simulink subsystem "tcp_trace_simscape_ref_subsys"  (R2022b)
settings: Solver=VariableStepAuto  StartTime=0.0  StopTime=10.0  RelTol=1e-3
undefined symbols (not defined in the file): param_vis
libraries: nesl_utility x300, sm_lib x200
(part 1 of 3)
settings Model: Creator=emu  LastModifiedBy=emu

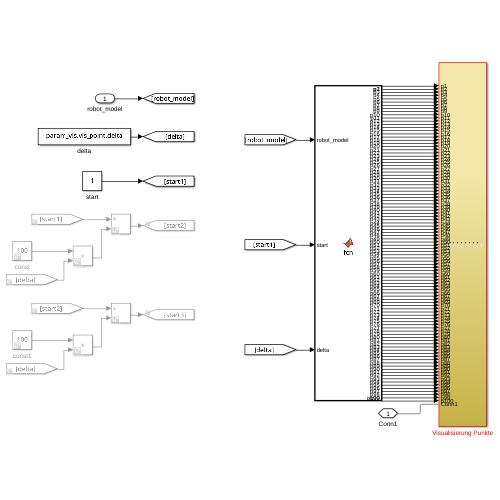
[thumbnail: Simulink's stored preview of the top-level diagram]
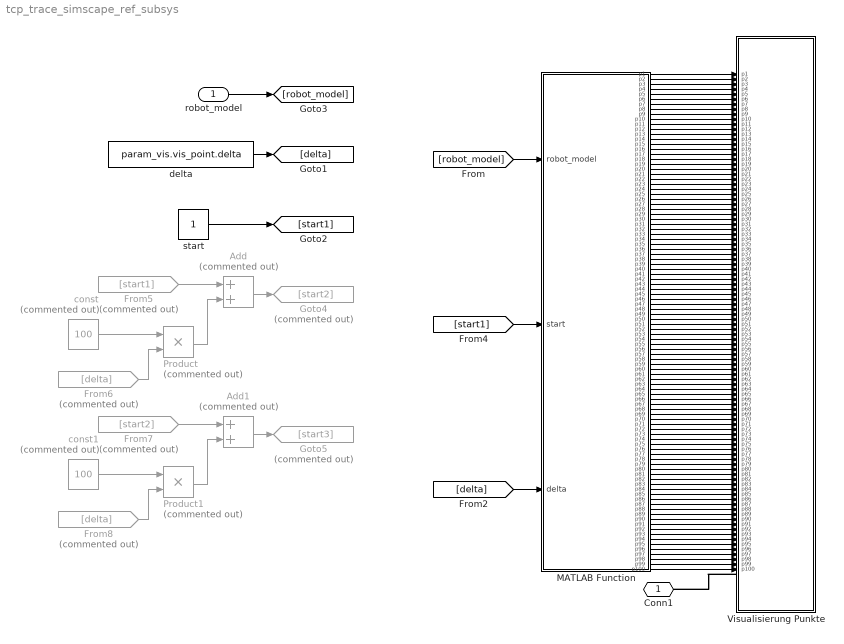
== system tcp_trace_simscape_ref_subsys ==
  robot_model : Inport
  Add : Sum  Commented=on
  Add1 : Sum  Commented=on
  From5 : From  Commented=on  GotoTag=start1
  From6 : From  Commented=on  GotoTag=delta
  From7 : From  Commented=on  GotoTag=start2
  From8 : From  Commented=on  GotoTag=delta
  Goto4 : Goto  Commented=on  GotoTag=start2
  Goto5 : Goto  Commented=on  GotoTag=start3
  MATLAB Function : MATLAB Function  TreatAsAtomicUnit=on
  Product : Product  Commented=on
  Product1 : Product  Commented=on
  Visualisierung Punkte : Subsystem
  const : Constant  Commented=on  Value=100
  const1 : Constant  Commented=on  Value=100
  delta : Constant  Value=param_vis.vis_point.delta
  start : Constant  SampleTime=-1
  Conn1 : PMIOPort  Side=Left
  wires:
  const1/1 -> Product1/1
  MATLAB Function/49(p49) -> Visualisierung Punkte/49(p49)
  Product1/1 -> Add1/2
  MATLAB Function/52(p52) -> Visualisierung Punkte/52(p52)
  MATLAB Function/98(p98) -> Visualisierung Punkte/98(p98)
  MATLAB Function/39(p39) -> Visualisierung Punkte/39(p39)
  MATLAB Function/19(p19) -> Visualisierung Punkte/19(p19)
  MATLAB Function/29(p29) -> Visualisierung Punkte/29(p29)
  MATLAB Function/24(p24) -> Visualisierung Punkte/24(p24)
  MATLAB Function/34(p34) -> Visualisierung Punkte/34(p34)
  MATLAB Function/40(p40) -> Visualisierung Punkte/40(p40)
  MATLAB Function/99(p99) -> Visualisierung Punkte/99(p99)
  MATLAB Function/20(p20) -> Visualisierung Punkte/20(p20)
  From7/1 -> Add1/1
  MATLAB Function/2(p2) -> Visualisierung Punkte/2(p2)
  MATLAB Function/74(p74) -> Visualisierung Punkte/74(p74)
  MATLAB Function/82(p82) -> Visualisierung Punkte/82(p82)
  MATLAB Function/30(p30) -> Visualisierung Punkte/30(p30)
  MATLAB Function/35(p35) -> Visualisierung Punkte/35(p35)
  MATLAB Function/25(p25) -> Visualisierung Punkte/25(p25)
  MATLAB Function/83(p83) -> Visualisierung Punkte/83(p83)
  MATLAB Function/57(p57) -> Visualisierung Punkte/57(p57)
  MATLAB Function/63(p63) -> Visualisierung Punkte/63(p63)
  MATLAB Function/41(p41) -> Visualisierung Punkte/41(p41)
  MATLAB Function/21(p21) -> Visualisierung Punkte/21(p21)
  MATLAB Function/100(p100) -> Visualisierung Punkte/100(p100)
  MATLAB Function/36(p36) -> Visualisierung Punkte/36(p36)
  MATLAB Function/26(p26) -> Visualisierung Punkte/26(p26)
  MATLAB Function/31(p31) -> Visualisierung Punkte/31(p31)
  MATLAB Function/17(p17) -> Visualisierung Punkte/17(p17)
  MATLAB Function/6(p6) -> Visualisierung Punkte/6(p6)
  MATLAB Function/46(p46) -> Visualisierung Punkte/46(p46)
  MATLAB Function/37(p37) -> Visualisierung Punkte/37(p37)
  MATLAB Function/32(p32) -> Visualisierung Punkte/32(p32)
  MATLAB Function/27(p27) -> Visualisierung Punkte/27(p27)
  [delta] -> MATLAB Function/3(delta)
  MATLAB Function/42(p42) -> Visualisierung Punkte/42(p42)
  MATLAB Function/22(p22) -> Visualisierung Punkte/22(p22)
  MATLAB Function/85(p85) -> Visualisierung Punkte/85(p85)
  MATLAB Function/67(p67) -> Visualisierung Punkte/67(p67)
  MATLAB Function/92(p92) -> Visualisierung Punkte/92(p92)
  MATLAB Function/11(p11) -> Visualisierung Punkte/11(p11)
  [start1] -> MATLAB Function/2(start)
  delta/1 -> [delta]
  MATLAB Function/10(p10) -> Visualisierung Punkte/10(p10)
  MATLAB Function/54(p54) -> Visualisierung Punkte/54(p54)
  MATLAB Function/86(p86) -> Visualisierung Punkte/86(p86)
  MATLAB Function/77(p77) -> Visualisierung Punkte/77(p77)
  MATLAB Function/16(p16) -> Visualisierung Punkte/16(p16)
  MATLAB Function/53(p53) -> Visualisierung Punkte/53(p53)
  From8/1 -> Product1/2
  MATLAB Function/38(p38) -> Visualisierung Punkte/38(p38)
  MATLAB Function/33(p33) -> Visualisierung Punkte/33(p33)
  MATLAB Function/28(p28) -> Visualisierung Punkte/28(p28)
  MATLAB Function/23(p23) -> Visualisierung Punkte/23(p23)
  MATLAB Function/59(p59) -> Visualisierung Punkte/59(p59)
  MATLAB Function/91(p91) -> Visualisierung Punkte/91(p91)
  From5/1 -> Add/1
  MATLAB Function/75(p75) -> Visualisierung Punkte/75(p75)
  MATLAB Function/73(p73) -> Visualisierung Punkte/73(p73)
  MATLAB Function/44(p44) -> Visualisierung Punkte/44(p44)
  MATLAB Function/4(p4) -> Visualisierung Punkte/4(p4)
  Add/1 -> Goto4/1
  MATLAB Function/97(p97) -> Visualisierung Punkte/97(p97)
  MATLAB Function/43(p43) -> Visualisierung Punkte/43(p43)
  MATLAB Function/18(p18) -> Visualisierung Punkte/18(p18)
  MATLAB Function/65(p65) -> Visualisierung Punkte/65(p65)
  MATLAB Function/81(p81) -> Visualisierung Punkte/81(p81)
  MATLAB Function/56(p56) -> Visualisierung Punkte/56(p56)
  MATLAB Function/72(p72) -> Visualisierung Punkte/72(p72)
  MATLAB Function/45(p45) -> Visualisierung Punkte/45(p45)
  MATLAB Function/5(p5) -> Visualisierung Punkte/5(p5)
  MATLAB Function/93(p93) -> Visualisierung Punkte/93(p93)
  Product/1 -> Add/2
  MATLAB Function/62(p62) -> Visualisierung Punkte/62(p62)
  const/1 -> Product/1
  MATLAB Function/78(p78) -> Visualisierung Punkte/78(p78)
  MATLAB Function/1(p1) -> Visualisierung Punkte/1(p1)
  From6/1 -> Product/2
  MATLAB Function/47(p47) -> Visualisierung Punkte/47(p47)
  MATLAB Function/7(p7) -> Visualisierung Punkte/7(p7)
  MATLAB Function/79(p79) -> Visualisierung Punkte/79(p79)
  MATLAB Function/9(p9) -> Visualisierung Punkte/9(p9)
  [robot_model] -> MATLAB Function/1(robot_model)
  MATLAB Function/88(p88) -> Visualisierung Punkte/88(p88)
  MATLAB Function/14(p14) -> Visualisierung Punkte/14(p14)
  MATLAB Function/66(p66) -> Visualisierung Punkte/66(p66)
  MATLAB Function/69(p69) -> Visualisierung Punkte/69(p69)
  MATLAB Function/12(p12) -> Visualisierung Punkte/12(p12)
  start/1 -> [start1]
  MATLAB Function/87(p87) -> Visualisierung Punkte/87(p87)
  MATLAB Function/50(p50) -> Visualisierung Punkte/50(p50)
  MATLAB Function/96(p96) -> Visualisierung Punkte/96(p96)
  MATLAB Function/90(p90) -> Visualisierung Punkte/90(p90)
  MATLAB Function/58(p58) -> Visualisierung Punkte/58(p58)
  MATLAB Function/89(p89) -> Visualisierung Punkte/89(p89)
  MATLAB Function/48(p48) -> Visualisierung Punkte/48(p48)
  MATLAB Function/8(p8) -> Visualisierung Punkte/8(p8)
  robot_model/1 -> [robot_model]
  MATLAB Function/13(p13) -> Visualisierung Punkte/13(p13)
  MATLAB Function/80(p80) -> Visualisierung Punkte/80(p80)
  MATLAB Function/70(p70) -> Visualisierung Punkte/70(p70)
  MATLAB Function/15(p15) -> Visualisierung Punkte/15(p15)
  MATLAB Function/3(p3) -> Visualisierung Punkte/3(p3)
  MATLAB Function/84(p84) -> Visualisierung Punkte/84(p84)
  MATLAB Function/76(p76) -> Visualisierung Punkte/76(p76)
  Add1/1 -> Goto5/1
  MATLAB Function/95(p95) -> Visualisierung Punkte/95(p95)
  MATLAB Function/94(p94) -> Visualisierung Punkte/94(p94)
  MATLAB Function/71(p71) -> Visualisierung Punkte/71(p71)
  MATLAB Function/55(p55) -> Visualisierung Punkte/55(p55)
  MATLAB Function/61(p61) -> Visualisierung Punkte/61(p61)
  MATLAB Function/64(p64) -> Visualisierung Punkte/64(p64)
  MATLAB Function/68(p68) -> Visualisierung Punkte/68(p68)
  MATLAB Function/60(p60) -> Visualisierung Punkte/60(p60)
  MATLAB Function/51(p51) -> Visualisierung Punkte/51(p51)
  connections:
  Visualisierung Punkte/LConn1 -- Conn1/RConn1

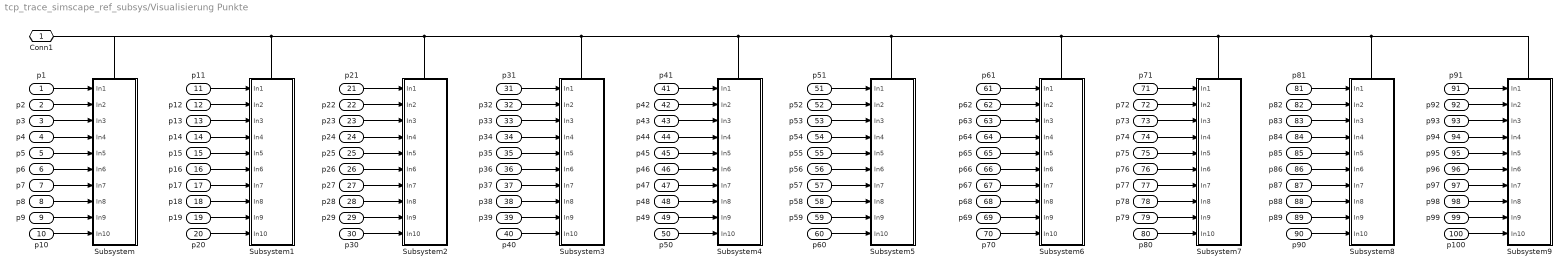
== system tcp_trace_simscape_ref_subsys/Visualisierung Punkte ==
  p1 : Inport
  p2 : Inport  Port=2
  p3 : Inport  Port=3
  p4 : Inport  Port=4
  p5 : Inport  Port=5
  p6 : Inport  Port=6
  p7 : Inport  Port=7
  p8 : Inport  Port=8
  p9 : Inport  Port=9
  p10 : Inport  Port=10
  p11 : Inport  Port=11
  p12 : Inport  Port=12
  p13 : Inport  Port=13
  p14 : Inport  Port=14
  p15 : Inport  Port=15
  p16 : Inport  Port=16
  p17 : Inport  Port=17
  p18 : Inport  Port=18
  p19 : Inport  Port=19
  p20 : Inport  Port=20
  p21 : Inport  Port=21
  p22 : Inport  Port=22
  p23 : Inport  Port=23
  p24 : Inport  Port=24
  p25 : Inport  Port=25
  p26 : Inport  Port=26
  p27 : Inport  Port=27
  p28 : Inport  Port=28
  p29 : Inport  Port=29
  p30 : Inport  Port=30
  p31 : Inport  Port=31
  p32 : Inport  Port=32
  p33 : Inport  Port=33
  p34 : Inport  Port=34
  p35 : Inport  Port=35
  p36 : Inport  Port=36
  p37 : Inport  Port=37
  p38 : Inport  Port=38
  p39 : Inport  Port=39
  p40 : Inport  Port=40
  p41 : Inport  Port=41
  p42 : Inport  Port=42
  p43 : Inport  Port=43
  p44 : Inport  Port=44
  p45 : Inport  Port=45
  p46 : Inport  Port=46
  p47 : Inport  Port=47
  p48 : Inport  Port=48
  p49 : Inport  Port=49
  p50 : Inport  Port=50
  p51 : Inport  Port=51
  p52 : Inport  Port=52
  p53 : Inport  Port=53
  p54 : Inport  Port=54
  p55 : Inport  Port=55
  p56 : Inport  Port=56
  p57 : Inport  Port=57
  p58 : Inport  Port=58
  p59 : Inport  Port=59
  p60 : Inport  Port=60
  p61 : Inport  Port=61
  p62 : Inport  Port=62
  p63 : Inport  Port=63
  p64 : Inport  Port=64
  p65 : Inport  Port=65
  p66 : Inport  Port=66
  p67 : Inport  Port=67
  p68 : Inport  Port=68
  p69 : Inport  Port=69
  p70 : Inport  Port=70
  p71 : Inport  Port=71
  p72 : Inport  Port=72
  p73 : Inport  Port=73
  p74 : Inport  Port=74
  p75 : Inport  Port=75
  p76 : Inport  Port=76
  p77 : Inport  Port=77
  p78 : Inport  Port=78
  p79 : Inport  Port=79
  p80 : Inport  Port=80
  p81 : Inport  Port=81
  p82 : Inport  Port=82
  p83 : Inport  Port=83
  p84 : Inport  Port=84
  p85 : Inport  Port=85
  p86 : Inport  Port=86
  p87 : Inport  Port=87
  p88 : Inport  Port=88
  p89 : Inport  Port=89
  p90 : Inport  Port=90
  p91 : Inport  Port=91
  p92 : Inport  Port=92
  p93 : Inport  Port=93
  p94 : Inport  Port=94
  p95 : Inport  Port=95
  p96 : Inport  Port=96
  p97 : Inport  Port=97
  p98 : Inport  Port=98
  p99 : Inport  Port=99
  p100 : Inport  Port=100
  Subsystem : Subsystem
      settings: PortSchema="{\"entries\":[{\"content\":{\"sides\":[{\"content\":{\"connectorIds\":[\"In1\",\"In2\",\"In3\",\"In4\",\"In5\",\"In6\",\"In7\",\"In8\",\"In9\",\"In10\"]},\"type\":\"ConnectorPlacement.EquallySpacedRectSide\",\"uuid\":\"2018066b-9524-48da-bbe6-ab202b76f720\"},{\"content\":{\"side\":\"RIGHT\"},\"type\":\"ConnectorPlacement.EquallySpacedRectSide\",\"uuid\":\"1983d9d9-cacf-48d4-9900-c1ea83df5447\"},{\"content\":{\"connectorIds\":[\"LConn1\"],\"side\":\"TOP\"},\"type\":\"ConnectorPlacement.EquallySpacedRectSide\",\"uuid\":\"d1112f51-9d46-44e1-99fb-55e38b45bdaf\"}]},\"type\":\"ConnectorPlacement.EquallySpacedConnector\",\"uuid\":\"be633077-5bce-4072-a8b6-d4330dd62166\"}],\"packageUris\":[\"http://schema.mathworks.com/mf0/Connector/R2020b\"],\"version\":\"1.0\"}"
  Subsystem1 : Subsystem
      settings: PortSchema="{\"entries\":[{\"content\":{\"sides\":[{\"content\":{\"connectorIds\":[\"In1\",\"In2\",\"In3\",\"In4\",\"In5\",\"In6\",\"In7\",\"In8\",\"In9\",\"In10\"]},\"type\":\"ConnectorPlacement.EquallySpacedRectSide\",\"uuid\":\"2018066b-9524-48da-bbe6-ab202b76f720\"},{\"content\":{\"side\":\"RIGHT\"},\"type\":\"ConnectorPlacement.EquallySpacedRectSide\",\"uuid\":\"1983d9d9-cacf-48d4-9900-c1ea83df5447\"},{\"content\":{\"connectorIds\":[\"LConn1\"],\"side\":\"TOP\"},\"type\":\"ConnectorPlacement.EquallySpacedRectSide\",\"uuid\":\"d1112f51-9d46-44e1-99fb-55e38b45bdaf\"}]},\"type\":\"ConnectorPlacement.EquallySpacedConnector\",\"uuid\":\"be633077-5bce-4072-a8b6-d4330dd62166\"}],\"packageUris\":[\"http://schema.mathworks.com/mf0/Connector/R2020b\"],\"version\":\"1.0\"}"
  Subsystem2 : Subsystem
      settings: PortSchema="{\"entries\":[{\"content\":{\"sides\":[{\"content\":{\"connectorIds\":[\"In1\",\"In2\",\"In3\",\"In4\",\"In5\",\"In6\",\"In7\",\"In8\",\"In9\",\"In10\"]},\"type\":\"ConnectorPlacement.EquallySpacedRectSide\",\"uuid\":\"2018066b-9524-48da-bbe6-ab202b76f720\"},{\"content\":{\"side\":\"RIGHT\"},\"type\":\"ConnectorPlacement.EquallySpacedRectSide\",\"uuid\":\"1983d9d9-cacf-48d4-9900-c1ea83df5447\"},{\"content\":{\"connectorIds\":[\"LConn1\"],\"side\":\"TOP\"},\"type\":\"ConnectorPlacement.EquallySpacedRectSide\",\"uuid\":\"d1112f51-9d46-44e1-99fb-55e38b45bdaf\"}]},\"type\":\"ConnectorPlacement.EquallySpacedConnector\",\"uuid\":\"be633077-5bce-4072-a8b6-d4330dd62166\"}],\"packageUris\":[\"http://schema.mathworks.com/mf0/Connector/R2020b\"],\"version\":\"1.0\"}"
  Subsystem3 : Subsystem
      settings: PortSchema="{\"entries\":[{\"content\":{\"sides\":[{\"content\":{\"connectorIds\":[\"In1\",\"In2\",\"In3\",\"In4\",\"In5\",\"In6\",\"In7\",\"In8\",\"In9\",\"In10\"]},\"type\":\"ConnectorPlacement.EquallySpacedRectSide\",\"uuid\":\"2018066b-9524-48da-bbe6-ab202b76f720\"},{\"content\":{\"side\":\"RIGHT\"},\"type\":\"ConnectorPlacement.EquallySpacedRectSide\",\"uuid\":\"1983d9d9-cacf-48d4-9900-c1ea83df5447\"},{\"content\":{\"connectorIds\":[\"LConn1\"],\"side\":\"TOP\"},\"type\":\"ConnectorPlacement.EquallySpacedRectSide\",\"uuid\":\"d1112f51-9d46-44e1-99fb-55e38b45bdaf\"}]},\"type\":\"ConnectorPlacement.EquallySpacedConnector\",\"uuid\":\"be633077-5bce-4072-a8b6-d4330dd62166\"}],\"packageUris\":[\"http://schema.mathworks.com/mf0/Connector/R2020b\"],\"version\":\"1.0\"}"
  Subsystem4 : Subsystem
      settings: PortSchema="{\"entries\":[{\"content\":{\"sides\":[{\"content\":{\"connectorIds\":[\"In1\",\"In2\",\"In3\",\"In4\",\"In5\",\"In6\",\"In7\",\"In8\",\"In9\",\"In10\"]},\"type\":\"ConnectorPlacement.EquallySpacedRectSide\",\"uuid\":\"2018066b-9524-48da-bbe6-ab202b76f720\"},{\"content\":{\"side\":\"RIGHT\"},\"type\":\"ConnectorPlacement.EquallySpacedRectSide\",\"uuid\":\"1983d9d9-cacf-48d4-9900-c1ea83df5447\"},{\"content\":{\"connectorIds\":[\"LConn1\"],\"side\":\"TOP\"},\"type\":\"ConnectorPlacement.EquallySpacedRectSide\",\"uuid\":\"d1112f51-9d46-44e1-99fb-55e38b45bdaf\"}]},\"type\":\"ConnectorPlacement.EquallySpacedConnector\",\"uuid\":\"be633077-5bce-4072-a8b6-d4330dd62166\"}],\"packageUris\":[\"http://schema.mathworks.com/mf0/Connector/R2020b\"],\"version\":\"1.0\"}"
  Subsystem5 : Subsystem
      settings: PortSchema="{\"entries\":[{\"content\":{\"sides\":[{\"content\":{\"connectorIds\":[\"In1\",\"In2\",\"In3\",\"In4\",\"In5\",\"In6\",\"In7\",\"In8\",\"In9\",\"In10\"]},\"type\":\"ConnectorPlacement.EquallySpacedRectSide\",\"uuid\":\"2018066b-9524-48da-bbe6-ab202b76f720\"},{\"content\":{\"side\":\"RIGHT\"},\"type\":\"ConnectorPlacement.EquallySpacedRectSide\",\"uuid\":\"1983d9d9-cacf-48d4-9900-c1ea83df5447\"},{\"content\":{\"connectorIds\":[\"LConn1\"],\"side\":\"TOP\"},\"type\":\"ConnectorPlacement.EquallySpacedRectSide\",\"uuid\":\"d1112f51-9d46-44e1-99fb-55e38b45bdaf\"}]},\"type\":\"ConnectorPlacement.EquallySpacedConnector\",\"uuid\":\"be633077-5bce-4072-a8b6-d4330dd62166\"}],\"packageUris\":[\"http://schema.mathworks.com/mf0/Connector/R2020b\"],\"version\":\"1.0\"}"
  Subsystem6 : Subsystem
      settings: PortSchema="{\"entries\":[{\"content\":{\"sides\":[{\"content\":{\"connectorIds\":[\"In1\",\"In2\",\"In3\",\"In4\",\"In5\",\"In6\",\"In7\",\"In8\",\"In9\",\"In10\"]},\"type\":\"ConnectorPlacement.EquallySpacedRectSide\",\"uuid\":\"2018066b-9524-48da-bbe6-ab202b76f720\"},{\"content\":{\"side\":\"RIGHT\"},\"type\":\"ConnectorPlacement.EquallySpacedRectSide\",\"uuid\":\"1983d9d9-cacf-48d4-9900-c1ea83df5447\"},{\"content\":{\"connectorIds\":[\"LConn1\"],\"side\":\"TOP\"},\"type\":\"ConnectorPlacement.EquallySpacedRectSide\",\"uuid\":\"d1112f51-9d46-44e1-99fb-55e38b45bdaf\"}]},\"type\":\"ConnectorPlacement.EquallySpacedConnector\",\"uuid\":\"be633077-5bce-4072-a8b6-d4330dd62166\"}],\"packageUris\":[\"http://schema.mathworks.com/mf0/Connector/R2020b\"],\"version\":\"1.0\"}"
  Subsystem7 : Subsystem
      settings: PortSchema="{\"entries\":[{\"content\":{\"sides\":[{\"content\":{\"connectorIds\":[\"In1\",\"In2\",\"In3\",\"In4\",\"In5\",\"In6\",\"In7\",\"In8\",\"In9\",\"In10\"]},\"type\":\"ConnectorPlacement.EquallySpacedRectSide\",\"uuid\":\"2018066b-9524-48da-bbe6-ab202b76f720\"},{\"content\":{\"side\":\"RIGHT\"},\"type\":\"ConnectorPlacement.EquallySpacedRectSide\",\"uuid\":\"1983d9d9-cacf-48d4-9900-c1ea83df5447\"},{\"content\":{\"connectorIds\":[\"LConn1\"],\"side\":\"TOP\"},\"type\":\"ConnectorPlacement.EquallySpacedRectSide\",\"uuid\":\"d1112f51-9d46-44e1-99fb-55e38b45bdaf\"}]},\"type\":\"ConnectorPlacement.EquallySpacedConnector\",\"uuid\":\"be633077-5bce-4072-a8b6-d4330dd62166\"}],\"packageUris\":[\"http://schema.mathworks.com/mf0/Connector/R2020b\"],\"version\":\"1.0\"}"
  Subsystem8 : Subsystem
      settings: PortSchema="{\"entries\":[{\"content\":{\"sides\":[{\"content\":{\"connectorIds\":[\"In1\",\"In2\",\"In3\",\"In4\",\"In5\",\"In6\",\"In7\",\"In8\",\"In9\",\"In10\"]},\"type\":\"ConnectorPlacement.EquallySpacedRectSide\",\"uuid\":\"2018066b-9524-48da-bbe6-ab202b76f720\"},{\"content\":{\"side\":\"RIGHT\"},\"type\":\"ConnectorPlacement.EquallySpacedRectSide\",\"uuid\":\"1983d9d9-cacf-48d4-9900-c1ea83df5447\"},{\"content\":{\"connectorIds\":[\"LConn1\"],\"side\":\"TOP\"},\"type\":\"ConnectorPlacement.EquallySpacedRectSide\",\"uuid\":\"d1112f51-9d46-44e1-99fb-55e38b45bdaf\"}]},\"type\":\"ConnectorPlacement.EquallySpacedConnector\",\"uuid\":\"be633077-5bce-4072-a8b6-d4330dd62166\"}],\"packageUris\":[\"http://schema.mathworks.com/mf0/Connector/R2020b\"],\"version\":\"1.0\"}"
  Subsystem9 : Subsystem
      settings: PortSchema="{\"entries\":[{\"content\":{\"sides\":[{\"content\":{\"connectorIds\":[\"In1\",\"In2\",\"In3\",\"In4\",\"In5\",\"In6\",\"In7\",\"In8\",\"In9\",\"In10\"]},\"type\":\"ConnectorPlacement.EquallySpacedRectSide\",\"uuid\":\"2018066b-9524-48da-bbe6-ab202b76f720\"},{\"content\":{\"side\":\"RIGHT\"},\"type\":\"ConnectorPlacement.EquallySpacedRectSide\",\"uuid\":\"1983d9d9-cacf-48d4-9900-c1ea83df5447\"},{\"content\":{\"connectorIds\":[\"LConn1\"],\"side\":\"TOP\"},\"type\":\"ConnectorPlacement.EquallySpacedRectSide\",\"uuid\":\"d1112f51-9d46-44e1-99fb-55e38b45bdaf\"}]},\"type\":\"ConnectorPlacement.EquallySpacedConnector\",\"uuid\":\"be633077-5bce-4072-a8b6-d4330dd62166\"}],\"packageUris\":[\"http://schema.mathworks.com/mf0/Connector/R2020b\"],\"version\":\"1.0\"}"
  Conn1 : PMIOPort  Side=Left
  wires:
  p1/1 -> Subsystem/1(In1)
  p2/1 -> Subsystem/2(In2)
  p3/1 -> Subsystem/3(In3)
  p4/1 -> Subsystem/4(In4)
  p5/1 -> Subsystem/5(In5)
  p6/1 -> Subsystem/6(In6)
  p7/1 -> Subsystem/7(In7)
  p8/1 -> Subsystem/8(In8)
  p9/1 -> Subsystem/9(In9)
  p10/1 -> Subsystem/10(In10)
  p20/1 -> Subsystem1/10(In10)
  p19/1 -> Subsystem1/9(In9)
  p18/1 -> Subsystem1/8(In8)
  p17/1 -> Subsystem1/7(In7)
  p16/1 -> Subsystem1/6(In6)
  p15/1 -> Subsystem1/5(In5)
  p14/1 -> Subsystem1/4(In4)
  p13/1 -> Subsystem1/3(In3)
  p12/1 -> Subsystem1/2(In2)
  p11/1 -> Subsystem1/1(In1)
  p21/1 -> Subsystem2/1(In1)
  p22/1 -> Subsystem2/2(In2)
  p23/1 -> Subsystem2/3(In3)
  p24/1 -> Subsystem2/4(In4)
  p25/1 -> Subsystem2/5(In5)
  p26/1 -> Subsystem2/6(In6)
  p27/1 -> Subsystem2/7(In7)
  p28/1 -> Subsystem2/8(In8)
  p29/1 -> Subsystem2/9(In9)
  p30/1 -> Subsystem2/10(In10)
  p60/1 -> Subsystem5/10(In10)
  p59/1 -> Subsystem5/9(In9)
  p58/1 -> Subsystem5/8(In8)
  p57/1 -> Subsystem5/7(In7)
  p56/1 -> Subsystem5/6(In6)
  p55/1 -> Subsystem5/5(In5)
  p54/1 -> Subsystem5/4(In4)
  p53/1 -> Subsystem5/3(In3)
  p52/1 -> Subsystem5/2(In2)
  p51/1 -> Subsystem5/1(In1)
  p41/1 -> Subsystem4/1(In1)
  p42/1 -> Subsystem4/2(In2)
  p43/1 -> Subsystem4/3(In3)
  p44/1 -> Subsystem4/4(In4)
  p45/1 -> Subsystem4/5(In5)
  p46/1 -> Subsystem4/6(In6)
  p47/1 -> Subsystem4/7(In7)
  p48/1 -> Subsystem4/8(In8)
  p49/1 -> Subsystem4/9(In9)
  p50/1 -> Subsystem4/10(In10)
  p40/1 -> Subsystem3/10(In10)
  p39/1 -> Subsystem3/9(In9)
  p38/1 -> Subsystem3/8(In8)
  p37/1 -> Subsystem3/7(In7)
  p36/1 -> Subsystem3/6(In6)
  p35/1 -> Subsystem3/5(In5)
  p34/1 -> Subsystem3/4(In4)
  p33/1 -> Subsystem3/3(In3)
  p32/1 -> Subsystem3/2(In2)
  p31/1 -> Subsystem3/1(In1)
  p61/1 -> Subsystem6/1(In1)
  p62/1 -> Subsystem6/2(In2)
  p63/1 -> Subsystem6/3(In3)
  p64/1 -> Subsystem6/4(In4)
  p65/1 -> Subsystem6/5(In5)
  p66/1 -> Subsystem6/6(In6)
  p67/1 -> Subsystem6/7(In7)
  p68/1 -> Subsystem6/8(In8)
  p69/1 -> Subsystem6/9(In9)
  p70/1 -> Subsystem6/10(In10)
  p80/1 -> Subsystem7/10(In10)
  p79/1 -> Subsystem7/9(In9)
  p78/1 -> Subsystem7/8(In8)
  p77/1 -> Subsystem7/7(In7)
  p76/1 -> Subsystem7/6(In6)
  p75/1 -> Subsystem7/5(In5)
  p74/1 -> Subsystem7/4(In4)
  p73/1 -> Subsystem7/3(In3)
  p72/1 -> Subsystem7/2(In2)
  p71/1 -> Subsystem7/1(In1)
  p81/1 -> Subsystem8/1(In1)
  p82/1 -> Subsystem8/2(In2)
  p83/1 -> Subsystem8/3(In3)
  p84/1 -> Subsystem8/4(In4)
  p85/1 -> Subsystem8/5(In5)
  p86/1 -> Subsystem8/6(In6)
  p87/1 -> Subsystem8/7(In7)
  p88/1 -> Subsystem8/8(In8)
  p89/1 -> Subsystem8/9(In9)
  p90/1 -> Subsystem8/10(In10)
  p100/1 -> Subsystem9/10(In10)
  p99/1 -> Subsystem9/9(In9)
  p98/1 -> Subsystem9/8(In8)
  p97/1 -> Subsystem9/7(In7)
  p96/1 -> Subsystem9/6(In6)
  p95/1 -> Subsystem9/5(In5)
  p94/1 -> Subsystem9/4(In4)
  p93/1 -> Subsystem9/3(In3)
  p92/1 -> Subsystem9/2(In2)
  p91/1 -> Subsystem9/1(In1)
  connections:
  Subsystem8/LConn1 -- Subsystem9/LConn1 -- Subsystem6/LConn1 -- Subsystem4/LConn1 -- Subsystem3/LConn1 -- Conn1/RConn1 -- Subsystem/LConn1 -- Subsystem1/LConn1 -- Subsystem2/LConn1 -- Subsystem5/LConn1 -- Subsystem7/LConn1

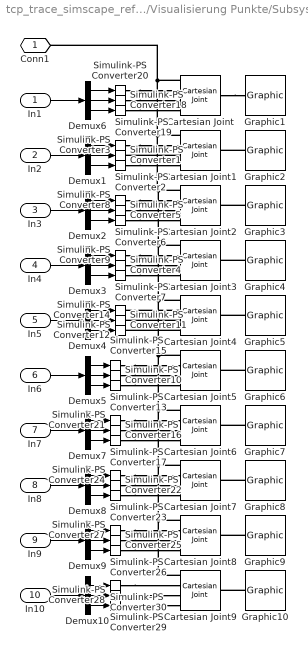
== system tcp_trace_simscape_ref_subsys/Visualisierung Punkte/Subsystem ==
  In1 : Inport
  In2 : Inport  Port=2
  In3 : Inport  Port=3
  In4 : Inport  Port=4
  In5 : Inport  Port=5
  In6 : Inport  Port=6
  In7 : Inport  Port=7
  In8 : Inport  Port=8
  In9 : Inport  Port=9
  In10 : Inport  Port=10
  Cartesian Joint{,1..9} (10 alike) : sm_lib/Joints/Cartesian Joint  JointMode=Normal  SenseConstraintForce=off  SenseConstraintForceX=off  SenseConstraintForceY=off  SenseConstraintForceZ=off  SenseConstraintTorque=off  SenseConstraintTorqueX=off  SenseConstraintTorqueY=off  SenseConstraintTorqueZ=off  SenseTotalForce=off  SenseTotalForceX=off  SenseTotalForceY=off  SenseTotalForceZ=off  SenseTotalTorque=off  SenseTotalTorqueX=off  SenseTotalTorqueY=off  SenseTotalTorqueZ=off  CompositeWrenchDir=FollowerOnBase  CompositeWrenchFrame=BaseFrame  PxEquilibriumPosition=0  PxEquilibriumPositionUnits=m  PxSpringStiffness=0  PxSpringStiffnessUnits=N/m  PxDampingCoefficient=0  PxDampingCoefficientUnits=N/(m/s)  PxTorqueActuationMode=ComputedTorque  PxMotionActuationMode=InputMotion  PxSensePosition=off  PxSenseVelocity=off  PxSenseAcceleration=off  PxSenseTorqueForce=off  PxSenseLowerLimitTorqueForce=off  PxSenseUpperLimitTorqueForce=off  PxLowerLimitSpecify=off  PxLowerLimitBound=-1  PxLowerLimitBoundUnits=m  PxLowerLimitStiffness=1e6  PxLowerLimitStiffnessUnits=N/m  PxLowerLimitDamping=1e3  PxLowerLimitDampingUnits=N/(m/s)  PxLowerLimitTransitionRegionWidth=1e-4  PxLowerLimitTransitionRegionWidthUnits=m  PxUpperLimitSpecify=off  PxUpperLimitBound=1  PxUpperLimitBoundUnits=m  PxUpperLimitStiffness=1e6  PxUpperLimitStiffnessUnits=N/m  PxUpperLimitDamping=1e3  PxUpperLimitDampingUnits=N/(m/s)  PxUpperLimitTransitionRegionWidth=1e-4  PxUpperLimitTransitionRegionWidthUnits=m  PxPositionTargetSpecify=off  PxPositionTargetPriority=High  PxPositionTargetValue=0  PxPositionTargetValueUnits=m  PxVelocityTargetSpecify=off  PxVelocityTargetPriority=High  PxVelocityTargetValue=0  PxVelocityTargetValueUnits=m/s  PyEquilibriumPosition=0  PyEquilibriumPositionUnits=m  PySpringStiffness=0  PySpringStiffnessUnits=N/m  PyDampingCoefficient=0  PyDampingCoefficientUnits=N/(m/s)  PyTorqueActuationMode=ComputedTorque  PyMotionActuationMode=InputMotion  PySensePosition=off  PySenseVelocity=off  PySenseAcceleration=off  PySenseTorqueForce=off  PySenseLowerLimitTorqueForce=off  PySenseUpperLimitTorqueForce=off  PyLowerLimitSpecify=off  PyLowerLimitBound=-1  PyLowerLimitBoundUnits=m  PyLowerLimitStiffness=1e6  PyLowerLimitStiffnessUnits=N/m  PyLowerLimitDamping=1e3  PyLowerLimitDampingUnits=N/(m/s)  PyLowerLimitTransitionRegionWidth=1e-4  PyLowerLimitTransitionRegionWidthUnits=m  PyUpperLimitSpecify=off  PyUpperLimitBound=1  PyUpperLimitBoundUnits=m  PyUpperLimitStiffness=1e6  PyUpperLimitStiffnessUnits=N/m  PyUpperLimitDamping=1e3  PyUpperLimitDampingUnits=N/(m/s)  PyUpperLimitTransitionRegionWidth=1e-4  PyUpperLimitTransitionRegionWidthUnits=m  PyPositionTargetSpecify=off  PyPositionTargetPriority=High  PyPositionTargetValue=0  PyPositionTargetValueUnits=m  PyVelocityTargetSpecify=off  PyVelocityTargetPriority=High  PyVelocityTargetValue=0  PyVelocityTargetValueUnits=m/s  PzEquilibriumPosition=0  PzEquilibriumPositionUnits=m  PzSpringStiffness=0  PzSpringStiffnessUnits=N/m  PzDampingCoefficient=0  PzDampingCoefficientUnits=N/(m/s)  PzTorqueActuationMode=ComputedTorque  PzMotionActuationMode=InputMotion  PzSensePosition=off  PzSenseVelocity=off  PzSenseAcceleration=off  PzSenseTorqueForce=off  PzSenseLowerLimitTorqueForce=off  PzSenseUpperLimitTorqueForce=off  PzLowerLimitSpecify=off  PzLowerLimitBound=-1  PzLowerLimitBoundUnits=m  PzLowerLimitStiffness=1e6  PzLowerLimitStiffnessUnits=N/m  PzLowerLimitDamping=1e3  PzLowerLimitDampingUnits=N/(m/s)  PzLowerLimitTransitionRegionWidth=1e-4  PzLowerLimitTransitionRegionWidthUnits=m  PzUpperLimitSpecify=off  PzUpperLimitBound=1  PzUpperLimitBoundUnits=m  PzUpperLimitStiffness=1e6  PzUpperLimitStiffnessUnits=N/m  PzUpperLimitDamping=1e3  PzUpperLimitDampingUnits=N/(m/s)  PzUpperLimitTransitionRegionWidth=1e-4  PzUpperLimitTransitionRegionWidthUnits=m  PzPositionTargetSpecify=off  PzPositionTargetPriority=High  PzPositionTargetValue=0  PzPositionTargetValueUnits=m  PzVelocityTargetSpecify=off  PzVelocityTargetPriority=High  PzVelocityTargetValue=0  PzVelocityTargetValueUnits=m/s
  Demux{1..10} (10 alike) : Demux  Outputs=3
  Graphic{1..10} (10 alike) : sm_lib/Body Elements/Graphic  GraphicType=Marker  MarkerShape=Sphere  MarkerSize=param_vis.vis_point.pix  GraphicVisPropType=SimpleVisualProperties  GraphicDiffuseColor=param_vis.vis_point.col  GraphicSpecularColor=[0.5 0.5 0.5 1.0]  GraphicAmbientColor=[0.15 0.15 0.15 1.0]  GraphicEmissiveColor=[0.0 0.0 0.0 1.0]  GraphicShininess=75  GraphicOpacity=param_vis.vis_point.opa
  Simulink-PS Converter{1..30} (30 alike) : nesl_utility/Simulink-PS Converter  PhysicalDomain=network_engine_domain  SubClassName=ps_input  LeftPortType=input  RightPortType=output  PseudoPeriodic=off  Frequencies=[]  NoiseDistribution=none  NoiseParameters=[]  Unit=1  AffineConversion=off  FilteringAndDerivatives=zero  SimscapeFilterOrder=2  InputFilterTimeConstant=0.001  UdotUserProvided=0
  Conn1 : PMIOPort  Side=Left
  wires:
  In7/1 -> Demux7/1
  In6/1 -> Demux5/1
  In10/1 -> Demux10/1
  In2/1 -> Demux1/1
  In5/1 -> Demux4/1
  In4/1 -> Demux3/1
  Demux6/3 -> Simulink-PS Converter19/1
  In3/1 -> Demux2/1
  In1/1 -> Demux6/1
  In9/1 -> Demux9/1
  In8/1 -> Demux8/1
  Demux6/1 -> Simulink-PS Converter20/1
  Demux6/2 -> Simulink-PS Converter18/1
  Demux1/1 -> Simulink-PS Converter3/1
  Demux4/2 -> Simulink-PS Converter11/1
  Demux4/1 -> Simulink-PS Converter14/1
  Demux4/3 -> Simulink-PS Converter12/1
  Demux1/2 -> Simulink-PS Converter1/1
  Demux1/3 -> Simulink-PS Converter2/1
  Demux2/1 -> Simulink-PS Converter8/1
  Demux2/2 -> Simulink-PS Converter5/1
  Demux2/3 -> Simulink-PS Converter6/1
  Demux3/3 -> Simulink-PS Converter7/1
  Demux3/1 -> Simulink-PS Converter9/1
  Demux3/2 -> Simulink-PS Converter4/1
  Demux5/1 -> Simulink-PS Converter15/1
  Demux5/2 -> Simulink-PS Converter10/1
  Demux5/3 -> Simulink-PS Converter13/1
  Demux7/1 -> Simulink-PS Converter21/1
  Demux7/2 -> Simulink-PS Converter16/1
  Demux7/3 -> Simulink-PS Converter17/1
  Demux8/1 -> Simulink-PS Converter24/1
  Demux8/2 -> Simulink-PS Converter22/1
  Demux8/3 -> Simulink-PS Converter23/1
  Demux9/1 -> Simulink-PS Converter27/1
  Demux9/2 -> Simulink-PS Converter25/1
  Demux9/3 -> Simulink-PS Converter26/1
  Demux10/1 -> Simulink-PS Converter30/1
  Demux10/2 -> Simulink-PS Converter28/1
  Demux10/3 -> Simulink-PS Converter29/1
  connections:
  Simulink-PS Converter19/RConn1 -- Cartesian Joint/LConn4
  Graphic4/RConn1 -- Cartesian Joint3/RConn1
  Cartesian Joint/RConn1 -- Graphic1/RConn1
  Graphic3/RConn1 -- Cartesian Joint2/RConn1
  Cartesian Joint8/LConn1 -- Cartesian Joint4/LConn1 -- Conn1/RConn1 -- Cartesian Joint/LConn1 -- Cartesian Joint1/LConn1 -- Cartesian Joint2/LConn1 -- Cartesian Joint3/LConn1 -- Cartesian Joint5/LConn1 -- Cartesian Joint6/LConn1 -- Cartesian Joint7/LConn1 -- Cartesian Joint9/LConn1
  Graphic7/RConn1 -- Cartesian Joint6/RConn1
  Graphic8/RConn1 -- Cartesian Joint7/RConn1
  Graphic6/RConn1 -- Cartesian Joint5/RConn1
  Graphic9/RConn1 -- Cartesian Joint8/RConn1
  Graphic2/RConn1 -- Cartesian Joint1/RConn1
  Graphic5/RConn1 -- Cartesian Joint4/RConn1
  Graphic10/RConn1 -- Cartesian Joint9/RConn1
  Simulink-PS Converter18/RConn1 -- Cartesian Joint/LConn3
  Simulink-PS Converter20/RConn1 -- Cartesian Joint/LConn2
  Simulink-PS Converter6/RConn1 -- Cartesian Joint2/LConn4
  Simulink-PS Converter8/RConn1 -- Cartesian Joint2/LConn2
  Simulink-PS Converter5/RConn1 -- Cartesian Joint2/LConn3
  Cartesian Joint4/LConn4 -- Simulink-PS Converter12/RConn1
  Cartesian Joint4/LConn2 -- Simulink-PS Converter14/RConn1
  Cartesian Joint4/LConn3 -- Simulink-PS Converter11/RConn1
  Simulink-PS Converter3/RConn1 -- Cartesian Joint1/LConn2
  Cartesian Joint1/LConn3 -- Simulink-PS Converter1/RConn1
  Simulink-PS Converter2/RConn1 -- Cartesian Joint1/LConn4
  Simulink-PS Converter15/RConn1 -- Cartesian Joint5/LConn2
  Simulink-PS Converter10/RConn1 -- Cartesian Joint5/LConn3
  Simulink-PS Converter13/RConn1 -- Cartesian Joint5/LConn4
  Simulink-PS Converter21/RConn1 -- Cartesian Joint6/LConn2
  Simulink-PS Converter16/RConn1 -- Cartesian Joint6/LConn3
  Simulink-PS Converter17/RConn1 -- Cartesian Joint6/LConn4
  Simulink-PS Converter24/RConn1 -- Cartesian Joint7/LConn2
  Simulink-PS Converter22/RConn1 -- Cartesian Joint7/LConn3
  Simulink-PS Converter23/RConn1 -- Cartesian Joint7/LConn4
  Simulink-PS Converter27/RConn1 -- Cartesian Joint8/LConn2
  Simulink-PS Converter25/RConn1 -- Cartesian Joint8/LConn3
  Simulink-PS Converter26/RConn1 -- Cartesian Joint8/LConn4
  Simulink-PS Converter30/RConn1 -- Cartesian Joint9/LConn2
  Simulink-PS Converter28/RConn1 -- Cartesian Joint9/LConn3
  Simulink-PS Converter29/RConn1 -- Cartesian Joint9/LConn4
  Simulink-PS Converter9/RConn1 -- Cartesian Joint3/LConn2
  Simulink-PS Converter4/RConn1 -- Cartesian Joint3/LConn3
  Simulink-PS Converter7/RConn1 -- Cartesian Joint3/LConn4

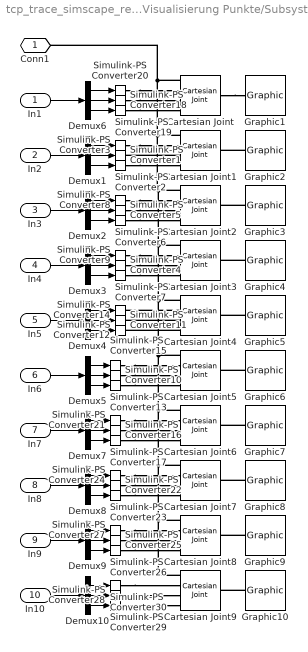
== system tcp_trace_simscape_ref_subsys/Visualisierung Punkte/Subsystem1 ==
  In1 : Inport
  In2 : Inport  Port=2
  In3 : Inport  Port=3
  In4 : Inport  Port=4
  In5 : Inport  Port=5
  In6 : Inport  Port=6
  In7 : Inport  Port=7
  In8 : Inport  Port=8
  In9 : Inport  Port=9
  In10 : Inport  Port=10
  Cartesian Joint{,1..9} (10 alike) : sm_lib/Joints/Cartesian Joint  JointMode=Normal  SenseConstraintForce=off  SenseConstraintForceX=off  SenseConstraintForceY=off  SenseConstraintForceZ=off  SenseConstraintTorque=off  SenseConstraintTorqueX=off  SenseConstraintTorqueY=off  SenseConstraintTorqueZ=off  SenseTotalForce=off  SenseTotalForceX=off  SenseTotalForceY=off  SenseTotalForceZ=off  SenseTotalTorque=off  SenseTotalTorqueX=off  SenseTotalTorqueY=off  SenseTotalTorqueZ=off  CompositeWrenchDir=FollowerOnBase  CompositeWrenchFrame=BaseFrame  PxEquilibriumPosition=0  PxEquilibriumPositionUnits=m  PxSpringStiffness=0  PxSpringStiffnessUnits=N/m  PxDampingCoefficient=0  PxDampingCoefficientUnits=N/(m/s)  PxTorqueActuationMode=ComputedTorque  PxMotionActuationMode=InputMotion  PxSensePosition=off  PxSenseVelocity=off  PxSenseAcceleration=off  PxSenseTorqueForce=off  PxSenseLowerLimitTorqueForce=off  PxSenseUpperLimitTorqueForce=off  PxLowerLimitSpecify=off  PxLowerLimitBound=-1  PxLowerLimitBoundUnits=m  PxLowerLimitStiffness=1e6  PxLowerLimitStiffnessUnits=N/m  PxLowerLimitDamping=1e3  PxLowerLimitDampingUnits=N/(m/s)  PxLowerLimitTransitionRegionWidth=1e-4  PxLowerLimitTransitionRegionWidthUnits=m  PxUpperLimitSpecify=off  PxUpperLimitBound=1  PxUpperLimitBoundUnits=m  PxUpperLimitStiffness=1e6  PxUpperLimitStiffnessUnits=N/m  PxUpperLimitDamping=1e3  PxUpperLimitDampingUnits=N/(m/s)  PxUpperLimitTransitionRegionWidth=1e-4  PxUpperLimitTransitionRegionWidthUnits=m  PxPositionTargetSpecify=off  PxPositionTargetPriority=High  PxPositionTargetValue=0  PxPositionTargetValueUnits=m  PxVelocityTargetSpecify=off  PxVelocityTargetPriority=High  PxVelocityTargetValue=0  PxVelocityTargetValueUnits=m/s  PyEquilibriumPosition=0  PyEquilibriumPositionUnits=m  PySpringStiffness=0  PySpringStiffnessUnits=N/m  PyDampingCoefficient=0  PyDampingCoefficientUnits=N/(m/s)  PyTorqueActuationMode=ComputedTorque  PyMotionActuationMode=InputMotion  PySensePosition=off  PySenseVelocity=off  PySenseAcceleration=off  PySenseTorqueForce=off  PySenseLowerLimitTorqueForce=off  PySenseUpperLimitTorqueForce=off  PyLowerLimitSpecify=off  PyLowerLimitBound=-1  PyLowerLimitBoundUnits=m  PyLowerLimitStiffness=1e6  PyLowerLimitStiffnessUnits=N/m  PyLowerLimitDamping=1e3  PyLowerLimitDampingUnits=N/(m/s)  PyLowerLimitTransitionRegionWidth=1e-4  PyLowerLimitTransitionRegionWidthUnits=m  PyUpperLimitSpecify=off  PyUpperLimitBound=1  PyUpperLimitBoundUnits=m  PyUpperLimitStiffness=1e6  PyUpperLimitStiffnessUnits=N/m  PyUpperLimitDamping=1e3  PyUpperLimitDampingUnits=N/(m/s)  PyUpperLimitTransitionRegionWidth=1e-4  PyUpperLimitTransitionRegionWidthUnits=m  PyPositionTargetSpecify=off  PyPositionTargetPriority=High  PyPositionTargetValue=0  PyPositionTargetValueUnits=m  PyVelocityTargetSpecify=off  PyVelocityTargetPriority=High  PyVelocityTargetValue=0  PyVelocityTargetValueUnits=m/s  PzEquilibriumPosition=0  PzEquilibriumPositionUnits=m  PzSpringStiffness=0  PzSpringStiffnessUnits=N/m  PzDampingCoefficient=0  PzDampingCoefficientUnits=N/(m/s)  PzTorqueActuationMode=ComputedTorque  PzMotionActuationMode=InputMotion  PzSensePosition=off  PzSenseVelocity=off  PzSenseAcceleration=off  PzSenseTorqueForce=off  PzSenseLowerLimitTorqueForce=off  PzSenseUpperLimitTorqueForce=off  PzLowerLimitSpecify=off  PzLowerLimitBound=-1  PzLowerLimitBoundUnits=m  PzLowerLimitStiffness=1e6  PzLowerLimitStiffnessUnits=N/m  PzLowerLimitDamping=1e3  PzLowerLimitDampingUnits=N/(m/s)  PzLowerLimitTransitionRegionWidth=1e-4  PzLowerLimitTransitionRegionWidthUnits=m  PzUpperLimitSpecify=off  PzUpperLimitBound=1  PzUpperLimitBoundUnits=m  PzUpperLimitStiffness=1e6  PzUpperLimitStiffnessUnits=N/m  PzUpperLimitDamping=1e3  PzUpperLimitDampingUnits=N/(m/s)  PzUpperLimitTransitionRegionWidth=1e-4  PzUpperLimitTransitionRegionWidthUnits=m  PzPositionTargetSpecify=off  PzPositionTargetPriority=High  PzPositionTargetValue=0  PzPositionTargetValueUnits=m  PzVelocityTargetSpecify=off  PzVelocityTargetPriority=High  PzVelocityTargetValue=0  PzVelocityTargetValueUnits=m/s
  Demux{1..10} (10 alike) : Demux  Outputs=3
  Graphic{1..10} (10 alike) : sm_lib/Body Elements/Graphic  GraphicType=Marker  MarkerShape=Sphere  MarkerSize=param_vis.vis_point.pix  GraphicVisPropType=SimpleVisualProperties  GraphicDiffuseColor=param_vis.vis_point.col  GraphicSpecularColor=[0.5 0.5 0.5 1.0]  GraphicAmbientColor=[0.15 0.15 0.15 1.0]  GraphicEmissiveColor=[0.0 0.0 0.0 1.0]  GraphicShininess=75  GraphicOpacity=param_vis.vis_point.opa
  Simulink-PS Converter{1..30} (30 alike) : nesl_utility/Simulink-PS Converter  PhysicalDomain=network_engine_domain  SubClassName=ps_input  LeftPortType=input  RightPortType=output  PseudoPeriodic=off  Frequencies=[]  NoiseDistribution=none  NoiseParameters=[]  Unit=1  AffineConversion=off  FilteringAndDerivatives=zero  SimscapeFilterOrder=2  InputFilterTimeConstant=0.001  UdotUserProvided=0
  Conn1 : PMIOPort  Side=Left
  wires:
  Demux10/3 -> Simulink-PS Converter29/1
  Demux10/2 -> Simulink-PS Converter28/1
  Demux10/1 -> Simulink-PS Converter30/1
  Demux9/3 -> Simulink-PS Converter26/1
  Demux9/2 -> Simulink-PS Converter25/1
  Demux9/1 -> Simulink-PS Converter27/1
  Demux8/3 -> Simulink-PS Converter23/1
  Demux8/2 -> Simulink-PS Converter22/1
  Demux8/1 -> Simulink-PS Converter24/1
  Demux7/3 -> Simulink-PS Converter17/1
  Demux7/2 -> Simulink-PS Converter16/1
  Demux7/1 -> Simulink-PS Converter21/1
  Demux5/3 -> Simulink-PS Converter13/1
  Demux5/2 -> Simulink-PS Converter10/1
  Demux5/1 -> Simulink-PS Converter15/1
  Demux3/2 -> Simulink-PS Converter4/1
  Demux3/1 -> Simulink-PS Converter9/1
  Demux3/3 -> Simulink-PS Converter7/1
  Demux2/3 -> Simulink-PS Converter6/1
  Demux2/2 -> Simulink-PS Converter5/1
  Demux2/1 -> Simulink-PS Converter8/1
  Demux1/3 -> Simulink-PS Converter2/1
  Demux1/2 -> Simulink-PS Converter1/1
  Demux4/3 -> Simulink-PS Converter12/1
  Demux4/1 -> Simulink-PS Converter14/1
  Demux4/2 -> Simulink-PS Converter11/1
  Demux1/1 -> Simulink-PS Converter3/1
  Demux6/2 -> Simulink-PS Converter18/1
  Demux6/1 -> Simulink-PS Converter20/1
  In8/1 -> Demux8/1
  In9/1 -> Demux9/1
  In1/1 -> Demux6/1
  In3/1 -> Demux2/1
  Demux6/3 -> Simulink-PS Converter19/1
  In4/1 -> Demux3/1
  In5/1 -> Demux4/1
  In2/1 -> Demux1/1
  In10/1 -> Demux10/1
  In6/1 -> Demux5/1
  In7/1 -> Demux7/1
  connections:
  Simulink-PS Converter7/RConn1 -- Cartesian Joint3/LConn4
  Simulink-PS Converter4/RConn1 -- Cartesian Joint3/LConn3
  Simulink-PS Converter9/RConn1 -- Cartesian Joint3/LConn2
  Simulink-PS Converter29/RConn1 -- Cartesian Joint9/LConn4
  Simulink-PS Converter28/RConn1 -- Cartesian Joint9/LConn3
  Simulink-PS Converter30/RConn1 -- Cartesian Joint9/LConn2
  Simulink-PS Converter26/RConn1 -- Cartesian Joint8/LConn4
  Simulink-PS Converter25/RConn1 -- Cartesian Joint8/LConn3
  Simulink-PS Converter27/RConn1 -- Cartesian Joint8/LConn2
  Simulink-PS Converter23/RConn1 -- Cartesian Joint7/LConn4
  Simulink-PS Converter22/RConn1 -- Cartesian Joint7/LConn3
  Simulink-PS Converter24/RConn1 -- Cartesian Joint7/LConn2
  Simulink-PS Converter17/RConn1 -- Cartesian Joint6/LConn4
  Simulink-PS Converter16/RConn1 -- Cartesian Joint6/LConn3
  Simulink-PS Converter21/RConn1 -- Cartesian Joint6/LConn2
  Simulink-PS Converter13/RConn1 -- Cartesian Joint5/LConn4
  Simulink-PS Converter10/RConn1 -- Cartesian Joint5/LConn3
  Simulink-PS Converter15/RConn1 -- Cartesian Joint5/LConn2
  Simulink-PS Converter2/RConn1 -- Cartesian Joint1/LConn4
  Cartesian Joint1/LConn3 -- Simulink-PS Converter1/RConn1
  Simulink-PS Converter3/RConn1 -- Cartesian Joint1/LConn2
  Cartesian Joint4/LConn3 -- Simulink-PS Converter11/RConn1
  Cartesian Joint4/LConn2 -- Simulink-PS Converter14/RConn1
  Cartesian Joint4/LConn4 -- Simulink-PS Converter12/RConn1
  Simulink-PS Converter5/RConn1 -- Cartesian Joint2/LConn3
  Simulink-PS Converter8/RConn1 -- Cartesian Joint2/LConn2
  Simulink-PS Converter6/RConn1 -- Cartesian Joint2/LConn4
  Simulink-PS Converter20/RConn1 -- Cartesian Joint/LConn2
  Simulink-PS Converter18/RConn1 -- Cartesian Joint/LConn3
  Graphic10/RConn1 -- Cartesian Joint9/RConn1
  Graphic5/RConn1 -- Cartesian Joint4/RConn1
  Graphic2/RConn1 -- Cartesian Joint1/RConn1
  Graphic9/RConn1 -- Cartesian Joint8/RConn1
  Graphic6/RConn1 -- Cartesian Joint5/RConn1
  Graphic8/RConn1 -- Cartesian Joint7/RConn1
  Graphic7/RConn1 -- Cartesian Joint6/RConn1
  Conn1/RConn1 -- Cartesian Joint/LConn1 -- Cartesian Joint1/LConn1 -- Cartesian Joint2/LConn1 -- Cartesian Joint3/LConn1 -- Cartesian Joint4/LConn1 -- Cartesian Joint5/LConn1 -- Cartesian Joint6/LConn1 -- Cartesian Joint7/LConn1 -- Cartesian Joint9/LConn1 -- Cartesian Joint8/LConn1
  Graphic3/RConn1 -- Cartesian Joint2/RConn1
  Cartesian Joint/RConn1 -- Graphic1/RConn1
  Graphic4/RConn1 -- Cartesian Joint3/RConn1
  Simulink-PS Converter19/RConn1 -- Cartesian Joint/LConn4

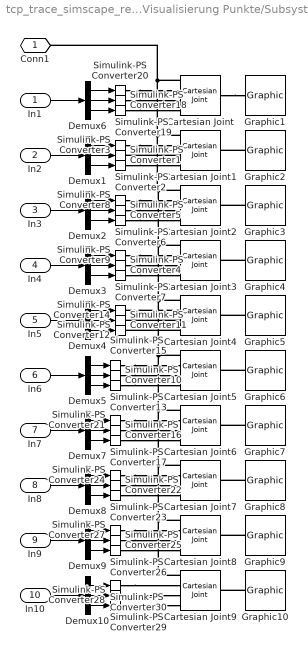
== system tcp_trace_simscape_ref_subsys/Visualisierung Punkte/Subsystem2 ==
  In1 : Inport
  In2 : Inport  Port=2
  In3 : Inport  Port=3
  In4 : Inport  Port=4
  In5 : Inport  Port=5
  In6 : Inport  Port=6
  In7 : Inport  Port=7
  In8 : Inport  Port=8
  In9 : Inport  Port=9
  In10 : Inport  Port=10
  Cartesian Joint{,1..9} (10 alike) : sm_lib/Joints/Cartesian Joint  JointMode=Normal  SenseConstraintForce=off  SenseConstraintForceX=off  SenseConstraintForceY=off  SenseConstraintForceZ=off  SenseConstraintTorque=off  SenseConstraintTorqueX=off  SenseConstraintTorqueY=off  SenseConstraintTorqueZ=off  SenseTotalForce=off  SenseTotalForceX=off  SenseTotalForceY=off  SenseTotalForceZ=off  SenseTotalTorque=off  SenseTotalTorqueX=off  SenseTotalTorqueY=off  SenseTotalTorqueZ=off  CompositeWrenchDir=FollowerOnBase  CompositeWrenchFrame=BaseFrame  PxEquilibriumPosition=0  PxEquilibriumPositionUnits=m  PxSpringStiffness=0  PxSpringStiffnessUnits=N/m  PxDampingCoefficient=0  PxDampingCoefficientUnits=N/(m/s)  PxTorqueActuationMode=ComputedTorque  PxMotionActuationMode=InputMotion  PxSensePosition=off  PxSenseVelocity=off  PxSenseAcceleration=off  PxSenseTorqueForce=off  PxSenseLowerLimitTorqueForce=off  PxSenseUpperLimitTorqueForce=off  PxLowerLimitSpecify=off  PxLowerLimitBound=-1  PxLowerLimitBoundUnits=m  PxLowerLimitStiffness=1e6  PxLowerLimitStiffnessUnits=N/m  PxLowerLimitDamping=1e3  PxLowerLimitDampingUnits=N/(m/s)  PxLowerLimitTransitionRegionWidth=1e-4  PxLowerLimitTransitionRegionWidthUnits=m  PxUpperLimitSpecify=off  PxUpperLimitBound=1  PxUpperLimitBoundUnits=m  PxUpperLimitStiffness=1e6  PxUpperLimitStiffnessUnits=N/m  PxUpperLimitDamping=1e3  PxUpperLimitDampingUnits=N/(m/s)  PxUpperLimitTransitionRegionWidth=1e-4  PxUpperLimitTransitionRegionWidthUnits=m  PxPositionTargetSpecify=off  PxPositionTargetPriority=High  PxPositionTargetValue=0  PxPositionTargetValueUnits=m  PxVelocityTargetSpecify=off  PxVelocityTargetPriority=High  PxVelocityTargetValue=0  PxVelocityTargetValueUnits=m/s  PyEquilibriumPosition=0  PyEquilibriumPositionUnits=m  PySpringStiffness=0  PySpringStiffnessUnits=N/m  PyDampingCoefficient=0  PyDampingCoefficientUnits=N/(m/s)  PyTorqueActuationMode=ComputedTorque  PyMotionActuationMode=InputMotion  PySensePosition=off  PySenseVelocity=off  PySenseAcceleration=off  PySenseTorqueForce=off  PySenseLowerLimitTorqueForce=off  PySenseUpperLimitTorqueForce=off  PyLowerLimitSpecify=off  PyLowerLimitBound=-1  PyLowerLimitBoundUnits=m  PyLowerLimitStiffness=1e6  PyLowerLimitStiffnessUnits=N/m  PyLowerLimitDamping=1e3  PyLowerLimitDampingUnits=N/(m/s)  PyLowerLimitTransitionRegionWidth=1e-4  PyLowerLimitTransitionRegionWidthUnits=m  PyUpperLimitSpecify=off  PyUpperLimitBound=1  PyUpperLimitBoundUnits=m  PyUpperLimitStiffness=1e6  PyUpperLimitStiffnessUnits=N/m  PyUpperLimitDamping=1e3  PyUpperLimitDampingUnits=N/(m/s)  PyUpperLimitTransitionRegionWidth=1e-4  PyUpperLimitTransitionRegionWidthUnits=m  PyPositionTargetSpecify=off  PyPositionTargetPriority=High  PyPositionTargetValue=0  PyPositionTargetValueUnits=m  PyVelocityTargetSpecify=off  PyVelocityTargetPriority=High  PyVelocityTargetValue=0  PyVelocityTargetValueUnits=m/s  PzEquilibriumPosition=0  PzEquilibriumPositionUnits=m  PzSpringStiffness=0  PzSpringStiffnessUnits=N/m  PzDampingCoefficient=0  PzDampingCoefficientUnits=N/(m/s)  PzTorqueActuationMode=ComputedTorque  PzMotionActuationMode=InputMotion  PzSensePosition=off  PzSenseVelocity=off  PzSenseAcceleration=off  PzSenseTorqueForce=off  PzSenseLowerLimitTorqueForce=off  PzSenseUpperLimitTorqueForce=off  PzLowerLimitSpecify=off  PzLowerLimitBound=-1  PzLowerLimitBoundUnits=m  PzLowerLimitStiffness=1e6  PzLowerLimitStiffnessUnits=N/m  PzLowerLimitDamping=1e3  PzLowerLimitDampingUnits=N/(m/s)  PzLowerLimitTransitionRegionWidth=1e-4  PzLowerLimitTransitionRegionWidthUnits=m  PzUpperLimitSpecify=off  PzUpperLimitBound=1  PzUpperLimitBoundUnits=m  PzUpperLimitStiffness=1e6  PzUpperLimitStiffnessUnits=N/m  PzUpperLimitDamping=1e3  PzUpperLimitDampingUnits=N/(m/s)  PzUpperLimitTransitionRegionWidth=1e-4  PzUpperLimitTransitionRegionWidthUnits=m  PzPositionTargetSpecify=off  PzPositionTargetPriority=High  PzPositionTargetValue=0  PzPositionTargetValueUnits=m  PzVelocityTargetSpecify=off  PzVelocityTargetPriority=High  PzVelocityTargetValue=0  PzVelocityTargetValueUnits=m/s
  Demux{1..10} (10 alike) : Demux  Outputs=3
  Graphic{1..10} (10 alike) : sm_lib/Body Elements/Graphic  GraphicType=Marker  MarkerShape=Sphere  MarkerSize=param_vis.vis_point.pix  GraphicVisPropType=SimpleVisualProperties  GraphicDiffuseColor=param_vis.vis_point.col  GraphicSpecularColor=[0.5 0.5 0.5 1.0]  GraphicAmbientColor=[0.15 0.15 0.15 1.0]  GraphicEmissiveColor=[0.0 0.0 0.0 1.0]  GraphicShininess=75  GraphicOpacity=param_vis.vis_point.opa
  Simulink-PS Converter{1..30} (30 alike) : nesl_utility/Simulink-PS Converter  PhysicalDomain=network_engine_domain  SubClassName=ps_input  LeftPortType=input  RightPortType=output  PseudoPeriodic=off  Frequencies=[]  NoiseDistribution=none  NoiseParameters=[]  Unit=1  AffineConversion=off  FilteringAndDerivatives=zero  SimscapeFilterOrder=2  InputFilterTimeConstant=0.001  UdotUserProvided=0
  Conn1 : PMIOPort  Side=Left
  wires:
  In7/1 -> Demux7/1
  In6/1 -> Demux5/1
  In10/1 -> Demux10/1
  In2/1 -> Demux1/1
  In5/1 -> Demux4/1
  In4/1 -> Demux3/1
  Demux6/3 -> Simulink-PS Converter19/1
  In3/1 -> Demux2/1
  In1/1 -> Demux6/1
  In9/1 -> Demux9/1
  In8/1 -> Demux8/1
  Demux6/1 -> Simulink-PS Converter20/1
  Demux6/2 -> Simulink-PS Converter18/1
  Demux1/1 -> Simulink-PS Converter3/1
  Demux4/2 -> Simulink-PS Converter11/1
  Demux4/1 -> Simulink-PS Converter14/1
  Demux4/3 -> Simulink-PS Converter12/1
  Demux1/2 -> Simulink-PS Converter1/1
  Demux1/3 -> Simulink-PS Converter2/1
  Demux2/1 -> Simulink-PS Converter8/1
  Demux2/2 -> Simulink-PS Converter5/1
  Demux2/3 -> Simulink-PS Converter6/1
  Demux3/3 -> Simulink-PS Converter7/1
  Demux3/1 -> Simulink-PS Converter9/1
  Demux3/2 -> Simulink-PS Converter4/1
  Demux5/1 -> Simulink-PS Converter15/1
  Demux5/2 -> Simulink-PS Converter10/1
  Demux5/3 -> Simulink-PS Converter13/1
  Demux7/1 -> Simulink-PS Converter21/1
  Demux7/2 -> Simulink-PS Converter16/1
  Demux7/3 -> Simulink-PS Converter17/1
  Demux8/1 -> Simulink-PS Converter24/1
  Demux8/2 -> Simulink-PS Converter22/1
  Demux8/3 -> Simulink-PS Converter23/1
  Demux9/1 -> Simulink-PS Converter27/1
  Demux9/2 -> Simulink-PS Converter25/1
  Demux9/3 -> Simulink-PS Converter26/1
  Demux10/1 -> Simulink-PS Converter30/1
  Demux10/2 -> Simulink-PS Converter28/1
  Demux10/3 -> Simulink-PS Converter29/1
  connections:
  Simulink-PS Converter19/RConn1 -- Cartesian Joint/LConn4
  Graphic4/RConn1 -- Cartesian Joint3/RConn1
  Cartesian Joint/RConn1 -- Graphic1/RConn1
  Graphic3/RConn1 -- Cartesian Joint2/RConn1
  Cartesian Joint8/LConn1 -- Cartesian Joint9/LConn1 -- Cartesian Joint7/LConn1 -- Cartesian Joint6/LConn1 -- Cartesian Joint5/LConn1 -- Cartesian Joint4/LConn1 -- Cartesian Joint3/LConn1 -- Cartesian Joint2/LConn1 -- Cartesian Joint1/LConn1 -- Cartesian Joint/LConn1 -- Conn1/RConn1
  Graphic7/RConn1 -- Cartesian Joint6/RConn1
  Graphic8/RConn1 -- Cartesian Joint7/RConn1
  Graphic6/RConn1 -- Cartesian Joint5/RConn1
  Graphic9/RConn1 -- Cartesian Joint8/RConn1
  Graphic2/RConn1 -- Cartesian Joint1/RConn1
  Graphic5/RConn1 -- Cartesian Joint4/RConn1
  Graphic10/RConn1 -- Cartesian Joint9/RConn1
  Simulink-PS Converter18/RConn1 -- Cartesian Joint/LConn3
  Simulink-PS Converter20/RConn1 -- Cartesian Joint/LConn2
  Simulink-PS Converter6/RConn1 -- Cartesian Joint2/LConn4
  Simulink-PS Converter8/RConn1 -- Cartesian Joint2/LConn2
  Simulink-PS Converter5/RConn1 -- Cartesian Joint2/LConn3
  Cartesian Joint4/LConn4 -- Simulink-PS Converter12/RConn1
  Cartesian Joint4/LConn2 -- Simulink-PS Converter14/RConn1
  Cartesian Joint4/LConn3 -- Simulink-PS Converter11/RConn1
  Simulink-PS Converter3/RConn1 -- Cartesian Joint1/LConn2
  Cartesian Joint1/LConn3 -- Simulink-PS Converter1/RConn1
  Simulink-PS Converter2/RConn1 -- Cartesian Joint1/LConn4
  Simulink-PS Converter15/RConn1 -- Cartesian Joint5/LConn2
  Simulink-PS Converter10/RConn1 -- Cartesian Joint5/LConn3
  Simulink-PS Converter13/RConn1 -- Cartesian Joint5/LConn4
  Simulink-PS Converter21/RConn1 -- Cartesian Joint6/LConn2
  Simulink-PS Converter16/RConn1 -- Cartesian Joint6/LConn3
  Simulink-PS Converter17/RConn1 -- Cartesian Joint6/LConn4
  Simulink-PS Converter24/RConn1 -- Cartesian Joint7/LConn2
  Simulink-PS Converter22/RConn1 -- Cartesian Joint7/LConn3
  Simulink-PS Converter23/RConn1 -- Cartesian Joint7/LConn4
  Simulink-PS Converter27/RConn1 -- Cartesian Joint8/LConn2
  Simulink-PS Converter25/RConn1 -- Cartesian Joint8/LConn3
  Simulink-PS Converter26/RConn1 -- Cartesian Joint8/LConn4
  Simulink-PS Converter30/RConn1 -- Cartesian Joint9/LConn2
  Simulink-PS Converter28/RConn1 -- Cartesian Joint9/LConn3
  Simulink-PS Converter29/RConn1 -- Cartesian Joint9/LConn4
  Simulink-PS Converter9/RConn1 -- Cartesian Joint3/LConn2
  Simulink-PS Converter4/RConn1 -- Cartesian Joint3/LConn3
  Simulink-PS Converter7/RConn1 -- Cartesian Joint3/LConn4
